simulink model "ADHW2p1"  (R2022a)
settings: Solver=VariableStepAuto  StartTime=0.0  StopTime=5400  RelTol=1e-3
settings Model: Creator=izacu  LastModifiedBy=izacu

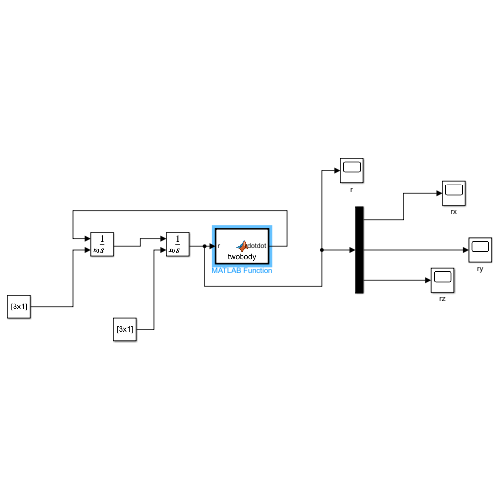
[thumbnail: Simulink's stored preview of the top-level diagram]
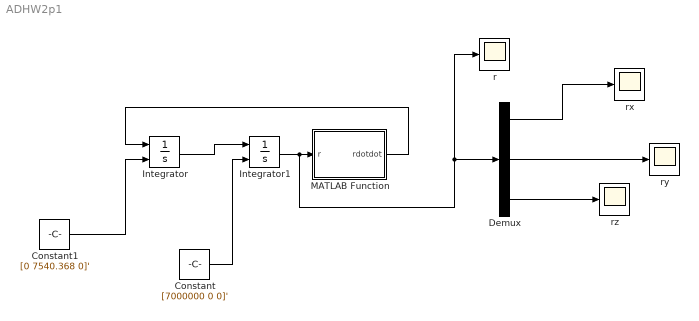
== system ADHW2p1 ==
  Constant : Constant  Value=[7000000 0 0]'  VectorParams1D=off
  Constant1 : Constant  Value=[0 7540.368 0]'
  Demux : Demux  Outputs=3
  Integrator : Integrator  InitialConditionSource=external
  Integrator1 : Integrator  InitialConditionSource=external
  MATLAB Function : MATLAB Function  TreatAsAtomicUnit=on
  r : Scope
  rx : Scope
  ry : Scope
  rz : Scope
  wires:
  Integrator/1 -> Integrator1/1
  Demux/1 -> rx/1
  Demux/3 -> rz/1
  Demux/2 -> ry/1
  Integrator1/1 -> r/1, Demux/1, MATLAB Function/1(r)
  MATLAB Function/1(rdotdot) -> Integrator/1
  Constant/1 -> Integrator1/2
  Constant1/1 -> Integrator/2

== matlab function ADHW2p1/MATLAB Function ==
  data: r input; rdotdot output
function rdotdot = twobody(r)
mu = 3.98E14;
rdotdot = (-mu.*r)./(norm(r)^3);
